simulink model "simulation"  (Simulink 8.7)
settings: Solver=VariableStepAuto  StartTime=0.0  StopTime=10.0  RelTol=1e-3
values from neighbouring files (symbols this model uses):
  A = [0 1 0 0; -k1/J1 -c1/J1 k1/J1 0;0 0 0 1; k1/J2 0 (-k1-k2)/J2 -c2/J2;]    [Controllable.m]    (also in ControllableV1.m = [0 1 0 0; ControllableV2.m = [0 1 0 0)
  B = [0; 1/J1; 0; 0;]    [Controllable.m]    (also in ControllableV1.m; ControllableV2.m)
  C = [1 0 0 0; 0 0 1 0]    [Controllable.m]    (also in ControllableV1.m = eye(4); ControllableV2.m = eye(4))
  D = [0;0]    [Controllable.m]    (also in ControllableV1.m = [0;0;0;0;]; ControllableV2.m = [0;0;0;0;])
  k = [k1 k2 k3 k4]    [Controllable.m]    (also in ControllableV1.m = kc / T; ControllableV2.m = kc / T)
settings Model: Creator=om_kha  LastModifiedBy=ramik
settings DataIOCC: LimitDataPoints=off  SaveFormat=Dataset
settings DebuggingCC: UnderspecifiedInitializationDetection=Simplified  MergeDetectMultiDrivingBlocksExec=error
settings HardwareCC: ProdBitPerPointer=64  ProdLargestAtomicFloat=Float  ProdIntDivRoundTo=Zero  ProdEndianess=LittleEndian  ProdWordSize=64  ProdHWDeviceType=Intel->x86-64 (Windows64)
settings ModelReferenceCC: PropagateSignalLabelsOutOfModel=on
settings ConfigComp: CovModelRefEnable=off

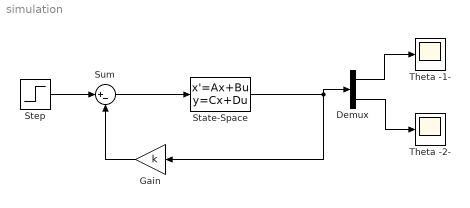
== system simulation ==
  Demux : Demux  Outputs=2
  Gain : Gain  Gain=k
  State-Space : StateSpace  A=A  B=B  C=C  D=D  X0=0  ContinuousStateAttributes=Situation
  Step : Step  SampleTime=0
  Sum : Sum  Inputs=|+-
  Theta -1- : Scope
  Theta -2- : Scope
  wires:
  Sum/1 -> State-Space/1
  State-Space/1 -> Demux/1, Gain/1
  Demux/1 -> Theta -1-/1
  Demux/2 -> Theta -2-/1
  Step/1 -> Sum/1
  Gain/1 -> Sum/2
